simulink model "MPAMBB_BER_binary"  (R2017a)
settings: Solver=VariableStepDiscrete  StartTime=0.0  StopTime=inf  RelTol=1e-3
values from neighbouring files (symbols this model uses):
  hrn = ones(1,OSF)/OSF    [scriptMPAMBB.m]
  M = 4    [scriptMPAMBB.m]
  OSF = 64    [scriptMPAMBB.m]
libraries: commdigbbndam3 x2, commchan3 x1, commrandsrc3 x1, commsink2 x1, commfilt2 x1, dspstat3 x1
settings Model: Creator=Fabio  LastModifiedBy=Fabio
settings DataIOCC: LimitDataPoints=on  SaveOutput=off  SaveTime=off
settings OptimizationCC: BooleanDataType=off  DefaultParameterBehavior=Inlined  LocalBlockOutputs=off  LifeSpan=inf
settings DebuggingCC: AlgebraicLoopMsg=error  SingleTaskRateTransMsg=error  AllowSymbolicDim=off  SFUnexpectedBacktrackingDiag=warning  SFNoUnconditionalDefaultTransitionDiag=warning  SFExecutionAtInitializationDiag=none
settings GRTTargetCC: TargetLangStandard=C89/C90 (ANSI)  GeneratePreprocessorConditionals=Disable all
settings ConfigComp: CovMetricSettings=dw  CovHtmlReporting=on  CovSaveCumulativeToWorkspaceVar=on  CovSaveSingleToWorkspaceVar=on  CovExternalEMLEnable=off  CovSFcnEnable=off

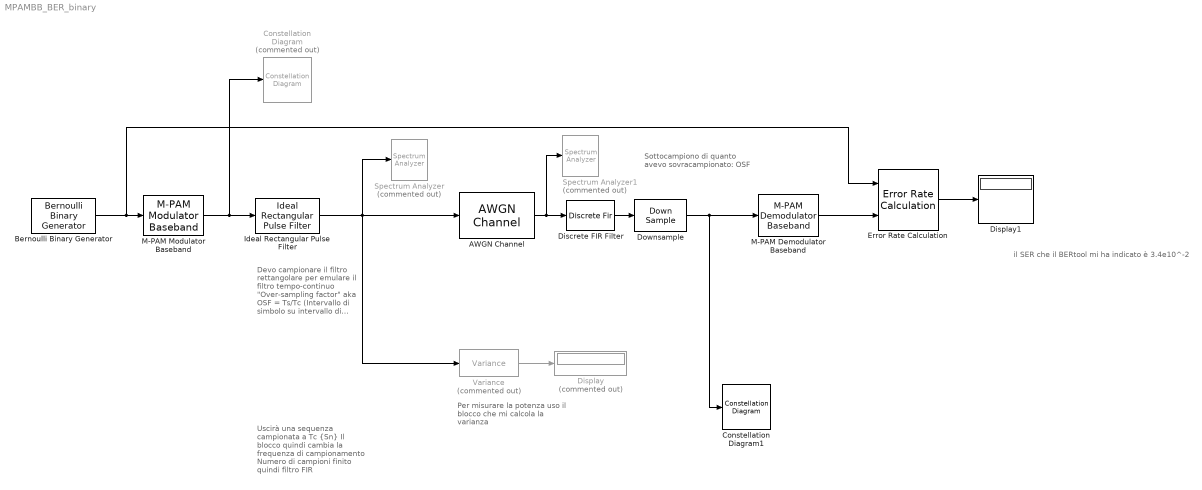
== system MPAMBB_BER_binary ==
  note: il SER che il BERtool mi ha indicato è 3.4e10^-2
  note: Sottocampiono di quanto avevo sovracampionato: OSF
  note: Per misurare la potenza uso il blocco che mi calcola la varianza
  note: Uscirà una sequenza campionata a Tc {Sn}
      | Il blocco quindi cambia la frequenza di campionamento
      | Numero di campioni finito quindi filtro FIR
  note: Devo campionare il filtro rettangolare
      | per emulare il filtro
      | tempo-continuo
      | "Over-sampling factor" aka OSF = Ts/Tc
      | (Intervallo di simbolo su intervallo di campionamento)
      | fc/Rs
      | quante volte campiono rispetto alla frequenza di simbolo
  AWGN Channel : commchan3/AWGN Channel  InputProcessing=Columns as channels (frame based)  seed=67  noiseMode="Signal to noise ratio  (Es/No)"  EbNodB=0.01  EsNodB=EbN0dB  SNRdB=10  bitsPerSym=1  Ps=(M^2 - 1)/3  Tsym=1  variance=1
  Bernoulli Binary Generator : commrandsrc3/Bernoulli Binary Generator  ProbabilityOfZero=0.5  SeedSource=Auto  Seed=0  SampleTime=1/log2(M)  SamplesPerFrame=log2(M)  OutputDataType=double  SimulateUsing=Interpreted execution
  Constellation Diagram : ConstellationDiagram  Commented=on
  Constellation Diagram1 : ConstellationDiagram
  Discrete FIR Filter : DiscreteFir  Coefficients=hrn  InputProcessing=Columns as channels (frame based)
  Display : Display  Commented=on
  Display1 : Display
  Downsample : DownSample  N=OSF  phase=OSF -1  RateOptions=Allow multirate processing
  Error Rate Calculation : commsink2/Error Rate Calculation  N=1  st_delay=0  cp_mode=Entire frame  subframe=[]  PMode=Port  WsName=ErrorVec  RsMode2=off  stop=off  numErr=100  maxBits=1e6
  Ideal Rectangular Pulse Filter : commfilt2/Ideal Rectangular Pulse Filter  pulseLen=OSF  pulseDelay=0  InputProcessing=Columns as channels (frame based)  RateOptions=Allow multirate processing  sampMode=Mute  normCheck=off  normMode=Sum of samples  filterGain=1  saveAsFlag=0  roundingMode=Floor  overflowMode=off  firstCoeffDataTypeStr=Inherit: Same word length as input  firstCoeffMin=[]  firstCoeffMax=[]  firstCoeffLastDataTypeStr=Inherit: Same word length as input  outputDataTypeStr=Inherit: Same as accumulator  outputMin=[]  outputMax=[]  outputLastDataTypeStr=Inherit: Same as accumulator
      settings: SourceProductName=Communications System Toolbox  SourceProductBaseCode=CM
  M-PAM Demodulator Baseband : commdigbbndam3/M-PAM Demodulator Baseband  M=M  OutType=Bit  Dec=Binary  PowType=Min. distance between symbols  MinDist=2  AvgPow=1  PeakPow=1  outDtype1=Inherit via internal rule  outDtype2=Inherit via internal rule  denormFactorWordLen=16  denormFactorDataTypeStr=Inherit: Same word length as input  denormFactorLastDataTypeStr=Inherit: Same word length as input  prodOutWordLen=16  prodOutRoundingMode=Floor  prodOutOverflowMode=Wrap  prodOutOvFlMode=off  prodOutOvFlModeLastStrValue=off  sumWordLen=16
      settings: SourceProductName=Communications System Toolbox  SourceProductBaseCode=CM
  M-PAM Modulator Baseband : commdigbbndam3/M-PAM Modulator Baseband  M=M  InType=Bit  Enc=Binary  PowType=Min. distance between symbols  MinDist=2  AvgPow=1  PeakPow=1  outDtype=double  outWordLen=16  outUDDataType=sfix(16)  outFracLenMode=Best precision  outFracLen=15  outDataTypeStr=double  outLastDataTypeStr=double
      settings: SourceProductName=Communications System Toolbox  SourceProductBaseCode=CM
  Spectrum Analyzer : SpectrumAnalyzer  Commented=on
  Spectrum Analyzer1 : SpectrumAnalyzer  Commented=on
  Variance : dspstat3/Variance  Commented=on  run=on  reset_popup=None  InputProcessing=Columns as channels (frame based)  directionMode=Each column  dimension=1  roiEnable=off  roiType=Rectangles  roiPortion=Entire ROI  roiOutput=Individual statistics for each ROI  roiFlag=off  roundingMode=Floor  overflowMode=off
      settings: SourceProductName=DSP System Toolbox
  wires:
  Bernoulli Binary Generator/1 -> Error Rate Calculation/1, M-PAM Modulator Baseband/1
  M-PAM Modulator Baseband/1 -> Constellation Diagram/1, Ideal Rectangular Pulse Filter/1
  Ideal Rectangular Pulse Filter/1 -> Variance/1, AWGN Channel/1, Spectrum Analyzer/1
  Variance/1 -> Display/1
  Discrete FIR Filter/1 -> Downsample/1
  Downsample/1 -> M-PAM Demodulator Baseband/1, Constellation Diagram1/1
  M-PAM Demodulator Baseband/1 -> Error Rate Calculation/2
  Error Rate Calculation/1 -> Display1/1
  AWGN Channel/1 -> Discrete FIR Filter/1, Spectrum Analyzer1/1
